simulink model "servo_dc_motor_sim_model"  (R2013b)
settings: Solver=ode45  StartTime=0.0  StopTime=0.6  RelTol=1e-3
libraries: powerlib x13, simulink x3, fl_lib x2
settings Model: Creator=User  LastModifiedBy=User
settings SolverCC: ZeroCrossControl=DisableAll

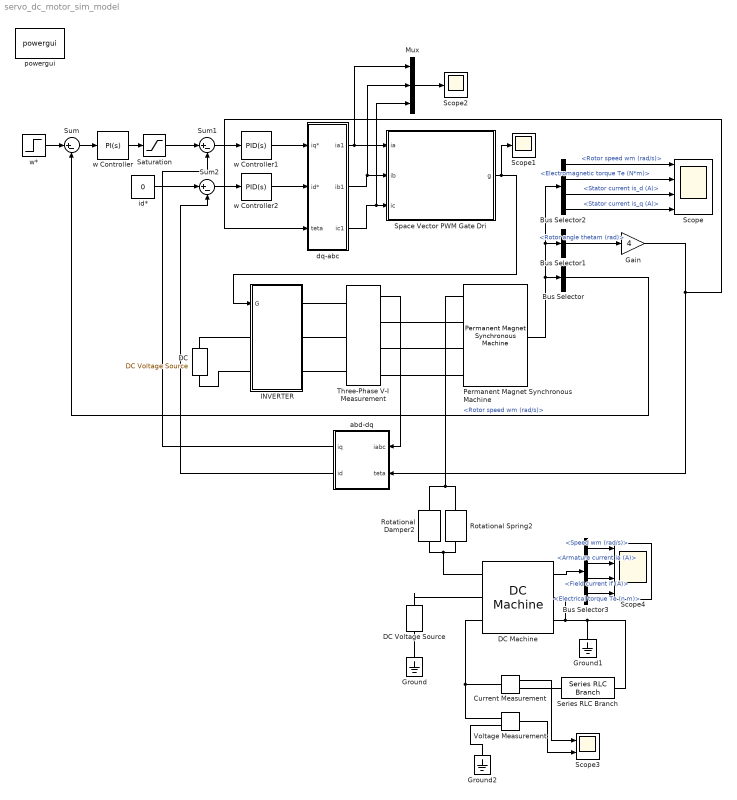
== system servo_dc_motor_sim_model ==
  Bus Selector : BusSelector  OutputSignals=Rotor speed wm (rad/s)
  Bus Selector1 : BusSelector  OutputSignals=Rotor angle thetam (rad)
  Bus Selector2 : BusSelector  OutputSignals=Rotor speed wm (rad/s),Electromagnetic torque Te (N*m),Stator current is_d (A),Stator current is_q (A)
  Bus Selector3 : BusSelector  OutputSignals=Speed wm (rad/s),Armature current ia (A),Field current if (A),Electrical torque Te (n m)
  Current Measurement : powerlib/Measurements/Current Measurement  PhasorSimulation=off  OutputType=Complex  PSBequivalent=0
  DC : powerlib/Electrical Sources/DC Voltage Source  Amplitude=400  Measurements=None
  DC Machine : powerlib/Machines/DC Machine  PresetModel=No  MechanicalLoad=Mechanical rotational port  FieldType=Wound  ShowDetailedParameters=on  RLa=[6.3 0.12]  RLf="[ 10.5  12]"  Laf=1.8  MachineConstant=Torque constant (N.m/A)  Ke=1.8  Kt=1.8  J=1  Bm=0  Tf=0  w0=1  Ifinit=1  TsPowergui=0  TsBlock=-1
  DC Voltage Source : powerlib/Electrical Sources/DC Voltage Source  Amplitude=12  Measurements=None
  Gain : Gain  Gain=4
  Ground : powerlib/Elements/Ground  LConnTagsString=a
  Ground1 : powerlib/Elements/Ground  LConnTagsString=a
  Ground2 : powerlib/Elements/Ground  LConnTagsString=a
  INVERTER : Subsystem
  Mux : Mux  Inputs=3
  Permanent Magnet Synchronous Machine : powerlib/Machines/Permanent Magnet Synchronous Machine  NbPhases=3  FluxDistribution=Sinusoidal  RotorType=Salient-pole  MechanicalLoad=Mechanical rotational port  PresetModel=No  ShowDetailedParameters=on  Resistance=0.61  Inductance=8.5e-3  dqInductances=[9.1e-3,11.5e-3]  La=0.000835  MachineConstant=Flux linkage established by magnets (V.s)  Flux=0.175  VoltageCst=126.966  TorqueCst=1.05  Flat=120  Mechanical=[0.0027 0.0004924 4 0]  PolePairs=4  InitialConditions=[0,0, 0,0]  InitialConditions5ph=[0 0 0 0 0 0]  TsPowergui=0  TsBlock=-1  RefAngle=90 degrees behind phase A axis (modified Park)
  Rotational Damper2 : fl_lib/Mechanical/Rotational Elements/Rotational Damper  D=1 N*m/(rad/s)  t_Log=off  w_Log=off  LocalVarNames=|t|w  LocalVarDescs=|t|w  LocalVarLogging=[0 0]
  Rotational Spring2 : fl_lib/Mechanical/Rotational Elements/Rotational Spring  spr_rate=5 N*m/rad  init_def=0 rad  t_Log=off  w_Log=off  phi_Log=off  LocalVarNames=|t|w|phi  LocalVarDescs=|t|w|phi  LocalVarLogging=[0 0 0]
  Saturation : Saturate  UpperLimit=20  LowerLimit=-20
  Scope : Scope  NumInputPorts=4
      settings: YMin=10~-25~-0.5~-20  YMax=110~25~7~20
  Scope1 : Scope
  Scope2 : Scope
      settings: YMin=-200  YMax=175  SaveName=ScopeData2
  Scope3 : Scope  NumInputPorts=2
      settings: YMin=-200~-5  YMax=175~5  SaveName=ScopeData5
  Scope4 : Scope  NumInputPorts=4
      settings: YMin=10~-25~-0.5~-20  YMax=110~25~7~20  SaveName=ScopeData6
  Series RLC Branch : powerlib/Elements/Series RLC Branch  LConnTagsString=__new0  RConnTagsString=__new0  BranchType=R  Resistance=20  Inductance=1e-3  SetiL0=off  InitialCurrent=0  Capacitance=1e-6  Setx0=off  InitialVoltage=0  Measurements=Branch voltage and current
  Space Vector PWM Gate Dri : Subsystem
  Sum : Sum  Inputs=|+-
  Sum1 : Sum  Inputs=|+-
  Sum2 : Sum  Inputs=|+-
  Three-Phase V-I Measurement : powerlib/Measurements/Three-Phase V-I Measurement  VoltageMeasurement=no  SetLabelV=off  LabelV=Vabc  Vpu=off  VpuLL=off  CurrentMeasurement=yes  SetLabelI=off  LabelI=Iabc  Ipu=off  Pbase=100e6  Vbase=500e3  OutputType=Complex  PhasorSimulation=off  PSBequivalent=0
  Voltage Measurement : powerlib/Measurements/Voltage Measurement  PhasorSimulation=off  OutputType=Complex  PSBequivalent=0
  abd-dq : Subsystem
  dq-abc : Subsystem
  id* : Constant  Value=0
  powergui : powerlib/powergui  Priority=1  SimulationMode=Continuous  SolverType=Tustin  SampleTime=50e-6  frequency=60  SPID=off  DisableSnubberDevices=off  DisableRonSwitches=off  DisableVfSwitches=off  SwTol=0  Interpol=off  DisplayEquations=off  frequencyindice=0  Pbase=100e6  ErrMax=1e-4  Iterations=50  UnitsV=kV  UnitsW=MW  FunctionMessages=off  echomessages=off  HookPort=off  EnableUseOfTLC=off  x0status=blocks  RestoreLinks=warning  ResistiveCurrentMeasurement=off  Frange=[0:2:500]  Ylog=off  Xlog=on  ShowGrid=off  save=off  variable=ZData  structure=ScopeData2  ZoomFFT=on  StartTime=0.05  cycles=10  DisplayStyle=1  fundamental=64.29  FreqAxis=on  MaxFrequency=1000  frequencyindicesteady=1  RmsSteady=1  display=off  Ts=0  methode=off
  w Controller : simulink/Continuous/PID Controller  Controller=PI  TimeDomain=Continuous-time  SampleTime=1  IntegratorMethod=Forward Euler  FilterMethod=Forward Euler  Form=Parallel  P=12  I=5  D=0  N=100  InitialConditionSource=internal  InitialConditionForIntegrator=0  InitialConditionForFilter=0  ExternalReset=none  LimitOutput=off  UpperSaturationLimit=inf  LowerSaturationLimit=-inf  LinearizeAsGain=on  AntiWindupMode=none  Kb=1  TrackingMode=off  Kt=1  PParamMin=[]  PParamMax=[]  IParamMin=[]  IParamMax=[]  DParamMin=[]  DParamMax=[]  NParamMin=[]  NParamMax=[]  KbParamMin=[]  KbParamMax=[]  KtParamMin=[]  KtParamMax=[]  POutMin=[]  POutMax=[]  IOutMin=[]  IOutMax=[]  DOutMin=[]  DOutMax=[]  NOutMin=[]  NOutMax=[]  KbOutMin=[]  KbOutMax=[]  KtOutMin=[]  KtOutMax=[]  IntegratorOutMin=[]  IntegratorOutMax=[]  FilterOutMin=[]  FilterOutMax=[]  SumOutMin=[]  SumOutMax=[]  SumI1OutMin=[]  SumI1OutMax=[]  SumI2OutMin=[]  SumI2OutMax=[]  SumI3OutMin=[]  SumI3OutMax=[]  SumDOutMin=[]  SumDOutMax=[]  SaturationOutMin=[]  SaturationOutMax=[]  IntegratorContinuousStateAttributes=''  IntegratorStateMustResolveToSignalObject=off  IntegratorRTWStateStorageClass=Auto  FilterContinuousStateAttributes=''  FilterStateMustResolveToSignalObject=off  FilterRTWStateStorageClass=Auto
  w Controller1 : simulink/Continuous/PID Controller  Controller=PID  TimeDomain=Continuous-time  SampleTime=1  IntegratorMethod=Forward Euler  FilterMethod=Forward Euler  Form=Parallel  P=5  I=12  D=5  N=100  InitialConditionSource=internal  InitialConditionForIntegrator=0  InitialConditionForFilter=0  ExternalReset=none  LimitOutput=off  UpperSaturationLimit=inf  LowerSaturationLimit=-inf  LinearizeAsGain=on  AntiWindupMode=none  Kb=1  TrackingMode=off  Kt=1  PParamMin=[]  PParamMax=[]  IParamMin=[]  IParamMax=[]  DParamMin=[]  DParamMax=[]  NParamMin=[]  NParamMax=[]  KbParamMin=[]  KbParamMax=[]  KtParamMin=[]  KtParamMax=[]  POutMin=[]  POutMax=[]  IOutMin=[]  IOutMax=[]  DOutMin=[]  DOutMax=[]  NOutMin=[]  NOutMax=[]  KbOutMin=[]  KbOutMax=[]  KtOutMin=[]  KtOutMax=[]  IntegratorOutMin=[]  IntegratorOutMax=[]  FilterOutMin=[]  FilterOutMax=[]  SumOutMin=[]  SumOutMax=[]  SumI1OutMin=[]  SumI1OutMax=[]  SumI2OutMin=[]  SumI2OutMax=[]  SumI3OutMin=[]  SumI3OutMax=[]  SumDOutMin=[]  SumDOutMax=[]  SaturationOutMin=[]  SaturationOutMax=[]  IntegratorContinuousStateAttributes=''  IntegratorStateMustResolveToSignalObject=off  IntegratorRTWStateStorageClass=Auto  FilterContinuousStateAttributes=''  FilterStateMustResolveToSignalObject=off  FilterRTWStateStorageClass=Auto
  w Controller2 : simulink/Continuous/PID Controller  Controller=PID  TimeDomain=Continuous-time  SampleTime=1  IntegratorMethod=Forward Euler  FilterMethod=Forward Euler  Form=Parallel  P=16  I=5  D=5  N=100  InitialConditionSource=internal  InitialConditionForIntegrator=0  InitialConditionForFilter=0  ExternalReset=none  LimitOutput=off  UpperSaturationLimit=inf  LowerSaturationLimit=-inf  LinearizeAsGain=on  AntiWindupMode=none  Kb=1  TrackingMode=off  Kt=1  PParamMin=[]  PParamMax=[]  IParamMin=[]  IParamMax=[]  DParamMin=[]  DParamMax=[]  NParamMin=[]  NParamMax=[]  KbParamMin=[]  KbParamMax=[]  KtParamMin=[]  KtParamMax=[]  POutMin=[]  POutMax=[]  IOutMin=[]  IOutMax=[]  DOutMin=[]  DOutMax=[]  NOutMin=[]  NOutMax=[]  KbOutMin=[]  KbOutMax=[]  KtOutMin=[]  KtOutMax=[]  IntegratorOutMin=[]  IntegratorOutMax=[]  FilterOutMin=[]  FilterOutMax=[]  SumOutMin=[]  SumOutMax=[]  SumI1OutMin=[]  SumI1OutMax=[]  SumI2OutMin=[]  SumI2OutMax=[]  SumI3OutMin=[]  SumI3OutMax=[]  SumDOutMin=[]  SumDOutMax=[]  SaturationOutMin=[]  SaturationOutMax=[]  IntegratorContinuousStateAttributes=''  IntegratorStateMustResolveToSignalObject=off  IntegratorRTWStateStorageClass=Auto  FilterContinuousStateAttributes=''  FilterStateMustResolveToSignalObject=off  FilterRTWStateStorageClass=Auto
  w* : Step  Time=0.3  Before=100  After=-100  SampleTime=0
  wires:
  Sum/1 -> w Controller/1
  w*/1 -> Sum/1
  Permanent Magnet Synchronous Machine/1 -> Bus Selector/1, Bus Selector1/1, Bus Selector2/1
  Bus Selector/1 -> Sum/2  "<Rotor speed wm (rad/s)>"
  Bus Selector1/1 -> Gain/1  "<Rotor angle thetam (rad)>"
  Bus Selector2/1 -> Scope/1  "<Rotor speed wm (rad/s)>"
  Bus Selector2/2 -> Scope/2  "<Electromagnetic torque Te (N*m)>"
  Bus Selector2/3 -> Scope/3  "<Stator current is_d (A)>"
  Bus Selector2/4 -> Scope/4  "<Stator current is_q (A)>"
  w Controller/1 -> Saturation/1
  Sum1/1 -> w Controller1/1
  w Controller1/1 -> dq-abc/1(iq*)
  id*/1 -> Sum2/1
  Sum2/1 -> w Controller2/1
  w Controller2/1 -> dq-abc/2(id*)
  Gain/1 -> abd-dq/2(teta), dq-abc/3(teta)
  Three-Phase V-I Measurement/1 -> abd-dq/1(iabc)
  abd-dq/1(iq) -> Sum1/2
  abd-dq/2(id) -> Sum2/2
  dq-abc/1(ia1) -> Mux/1, Space Vector PWM Gate Dri/1(ia)
  dq-abc/2(ib1) -> Mux/2, Space Vector PWM Gate Dri/2(ib)
  dq-abc/3(ic1) -> Mux/3, Space Vector PWM Gate Dri/3(ic)
  Space Vector PWM Gate Dri/1(g) -> INVERTER/1(G), Scope1/1
  Mux/1 -> Scope2/1
  Saturation/1 -> Sum1/1
  Current Measurement/1 -> Scope3/1
  Voltage Measurement/1 -> Scope3/2
  DC Machine/1 -> Bus Selector3/1
  Bus Selector3/1 -> Scope4/1  "<Speed wm (rad/s)>"
  Bus Selector3/2 -> Scope4/2  "<Armature current ia (A)>"
  Bus Selector3/3 -> Scope4/3  "<Field current if (A)>"
  Bus Selector3/4 -> Scope4/4  "<Electrical torque Te (n m)>"
  connections:
  Three-Phase V-I Measurement/LConn1 -- INVERTER/RConn1
  Three-Phase V-I Measurement/LConn2 -- INVERTER/RConn2
  Three-Phase V-I Measurement/LConn3 -- INVERTER/RConn3
  Three-Phase V-I Measurement/RConn1 -- Permanent Magnet Synchronous Machine/LConn2
  Three-Phase V-I Measurement/RConn2 -- Permanent Magnet Synchronous Machine/LConn3
  Three-Phase V-I Measurement/RConn3 -- Permanent Magnet Synchronous Machine/LConn4
  DC/RConn1 -- INVERTER/LConn1
  DC/LConn1 -- INVERTER/LConn2
  Rotational Spring2/RConn1 -- DC Machine/LConn1 -- Rotational Damper2/RConn1
  Rotational Damper2/LConn1 -- Permanent Magnet Synchronous Machine/LConn1 -- Rotational Spring2/LConn1
  DC Voltage Source/RConn1 -- DC Machine/LConn2
  Ground/LConn1 -- DC Voltage Source/LConn1
  Series RLC Branch/RConn1 -- DC Machine/RConn1 -- DC Machine/RConn2 -- Ground1/LConn1
  Current Measurement/RConn1 -- Series RLC Branch/LConn1
  DC Machine/LConn3 -- Voltage Measurement/LConn1 -- Current Measurement/LConn1
  Voltage Measurement/LConn2 -- Ground2/LConn1

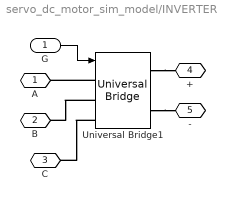
== system servo_dc_motor_sim_model/INVERTER ==
  G : Inport
  Universal Bridge1 : powerlib/Power Electronics/Universal Bridge  Arms=3  SnubberResistance=1e5  SnubberCapacitance=inf  Device=IGBT / Diodes  Ron=1e-3  Lon=0  ForwardVoltages="[  0  0  ]"  ForwardVoltage=0  GTOparameters=[ 10e-6 , 20e-6 ]  IGBTparameters=[ 1e-6 , 2e-6 ]  Measurements=None  Measurements_2=None  converterType=Rectifier
  A : PMIOPort  Port=1  Side=Right
  B : PMIOPort  Port=2  Side=Right
  C : PMIOPort  Port=3  Side=Right
  + : PMIOPort  Port=4  Side=Left
  - : PMIOPort  Port=5  Side=Left
  wires:
  G/1 -> Universal Bridge1/1
  connections:
  Universal Bridge1/RConn2 -- -/RConn1
  Universal Bridge1/RConn1 -- +/RConn1
  Universal Bridge1/LConn3 -- C/RConn1
  Universal Bridge1/LConn2 -- B/RConn1
  Universal Bridge1/LConn1 -- A/RConn1

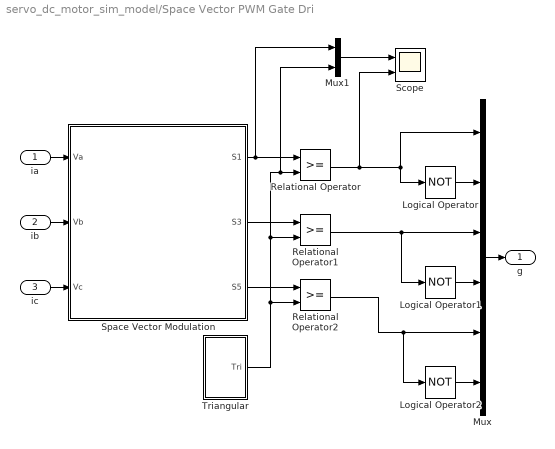
== system servo_dc_motor_sim_model/Space Vector PWM Gate Dri ==
  ia : Inport
  ib : Inport  Port=2
  ic : Inport  Port=3
  Logical Operator : Logic  Operator=NOT  AllPortsSameDT=off  OutDataTypeStr=boolean
  Logical Operator1 : Logic  Operator=NOT  AllPortsSameDT=off  OutDataTypeStr=boolean
  Logical Operator2 : Logic  Operator=NOT  AllPortsSameDT=off  OutDataTypeStr=boolean
  Mux : Mux  Inputs=6
  Mux1 : Mux  Inputs=2
  Relational Operator : RelationalOperator  OutDataTypeStr=boolean
  Relational Operator1 : RelationalOperator  OutDataTypeStr=boolean
  Relational Operator2 : RelationalOperator  OutDataTypeStr=boolean
  Scope : Scope  NumInputPorts=2
      settings: YMin=-0.05~0.95  YMax=1.05~1.05  SaveName=ScopeData4
  Space Vector Modulation : Subsystem
  Triangular : Subsystem
  g : Outport
  wires:
  Logical Operator/1 -> Mux/2
  Relational Operator1/1 -> Logical Operator1/1, Mux/3
  Triangular/1(Tri) -> Relational Operator2/2, Relational Operator1/2, Mux1/2, Relational Operator/2
  Space Vector Modulation/1(S1) -> Mux1/1, Relational Operator/1
  Space Vector Modulation/2(S3) -> Relational Operator1/1
  Space Vector Modulation/3(S5) -> Relational Operator2/1
  Mux/1 -> g/1
  Relational Operator/1 -> Scope/2, Logical Operator/1, Mux/1
  ia/1 -> Space Vector Modulation/1(Va)
  Logical Operator1/1 -> Mux/4
  Logical Operator2/1 -> Mux/6
  Relational Operator2/1 -> Logical Operator2/1, Mux/5
  ib/1 -> Space Vector Modulation/2(Vb)
  ic/1 -> Space Vector Modulation/3(Vc)
  Mux1/1 -> Scope/1

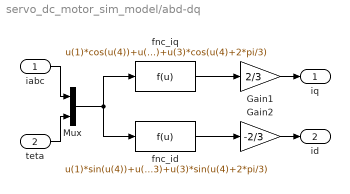
== system servo_dc_motor_sim_model/abd-dq ==
  iabc : Inport
  teta : Inport  Port=2
  Gain1 : Gain  Gain=2/3
  Gain2 : Gain  Gain=-2/3
  Mux : Mux  Inputs=2
  fnc_id : Fcn  Expr=u(1)*sin(u(4))+u(2)*sin(u(4)-2*pi/3)+u(3)*sin(u(4)+2*pi/3)
  fnc_iq : Fcn  Expr=u(1)*cos(u(4))+u(2)*cos(u(4)-2*pi/3)+u(3)*cos(u(4)+2*pi/3)
  iq : Outport
  id : Outport  Port=2
  wires:
  fnc_id/1 -> Gain2/1
  Gain1/1 -> iq/1
  teta/1 -> Mux/2
  iabc/1 -> Mux/1
  Mux/1 -> fnc_iq/1, fnc_id/1
  Gain2/1 -> id/1
  fnc_iq/1 -> Gain1/1

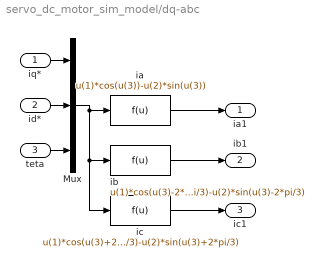
== system servo_dc_motor_sim_model/dq-abc ==
  iq* : Inport
  id* : Inport  Port=2
  teta : Inport  Port=3
  Mux : Mux  Inputs=3
  ia : Fcn  Expr=u(1)*cos(u(3))-u(2)*sin(u(3))
  ib : Fcn  Expr=u(1)*cos(u(3)-2*pi/3)-u(2)*sin(u(3)-2*pi/3)
  ic : Fcn  Expr=u(1)*cos(u(3)+2*pi/3)-u(2)*sin(u(3)+2*pi/3)
  ia1 : Outport
  ib1 : Outport  Port=2
  ic1 : Outport  Port=3
  wires:
  id*/1 -> Mux/2
  ia/1 -> ia1/1
  ib/1 -> ib1/1
  teta/1 -> Mux/3
  ic/1 -> ic1/1
  iq*/1 -> Mux/1
  Mux/1 -> ic/1, ib/1, ia/1

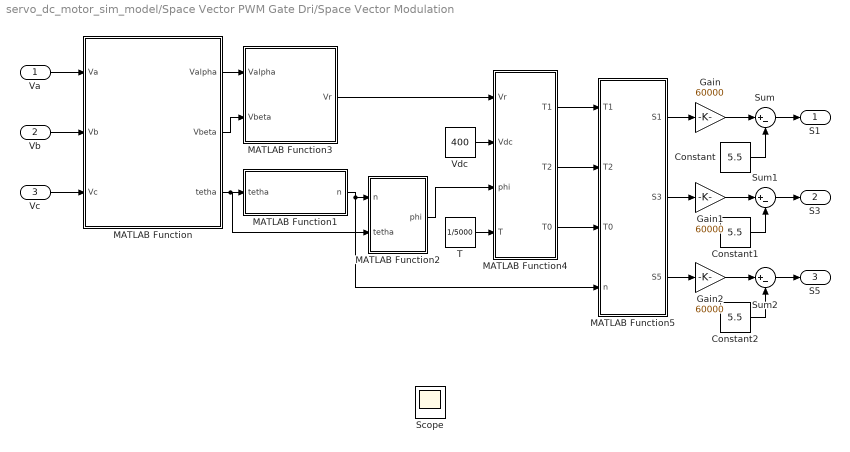
== system servo_dc_motor_sim_model/Space Vector PWM Gate Dri/Space Vector Modulation ==
  Va : Inport
  Vb : Inport  Port=2
  Vc : Inport  Port=3
  Constant : Constant  Value=5.5
  Constant1 : Constant  Value=5.5
  Constant2 : Constant  Value=5.5
  Gain : Gain  Gain=60000
  Gain1 : Gain  Gain=60000
  Gain2 : Gain  Gain=60000
  MATLAB Function : MATLAB Function  TreatAsAtomicUnit=on
  MATLAB Function1 : MATLAB Function  TreatAsAtomicUnit=on
  MATLAB Function2 : MATLAB Function  TreatAsAtomicUnit=on
  MATLAB Function3 : MATLAB Function  TreatAsAtomicUnit=on
  MATLAB Function4 : MATLAB Function  TreatAsAtomicUnit=on
  MATLAB Function5 : MATLAB Function  TreatAsAtomicUnit=on
  Scope : Scope
      settings: SaveName=ScopeData3
  Sum : Sum  Inputs=|+-
  Sum1 : Sum  Inputs=|+-
  Sum2 : Sum  Inputs=|+-
  T : Constant  Value=1/5000
  Vdc : Constant  Value=400
  S1 : Outport
  S3 : Outport  Port=2
  S5 : Outport  Port=3
  wires:
  MATLAB Function4/1(T1) -> MATLAB Function5/1(T1)
  MATLAB Function5/3(S5) -> Gain2/1
  MATLAB Function5/1(S1) -> Gain/1
  MATLAB Function4/2(T2) -> MATLAB Function5/2(T2)
  MATLAB Function4/3(T0) -> MATLAB Function5/3(T0)
  Va/1 -> MATLAB Function/1(Va)
  Vc/1 -> MATLAB Function/3(Vc)
  Vb/1 -> MATLAB Function/2(Vb)
  MATLAB Function/3(tetha) -> MATLAB Function2/2(tetha), MATLAB Function1/1(tetha)
  MATLAB Function1/1(n) -> MATLAB Function5/4(n), MATLAB Function2/1(n)
  MATLAB Function/1(Valpha) -> MATLAB Function3/1(Valpha)
  MATLAB Function/2(Vbeta) -> MATLAB Function3/2(Vbeta)
  MATLAB Function2/1(phi) -> MATLAB Function4/3(phi)
  MATLAB Function3/1(Vr) -> MATLAB Function4/1(Vr)
  Vdc/1 -> MATLAB Function4/2(Vdc)
  T/1 -> MATLAB Function4/4(T)
  MATLAB Function5/2(S3) -> Gain1/1
  Constant/1 -> Sum/2
  Gain/1 -> Sum/1
  Sum/1 -> S1/1
  Constant2/1 -> Sum2/2
  Constant1/1 -> Sum1/2
  Gain1/1 -> Sum1/1
  Sum1/1 -> S3/1
  Sum2/1 -> S5/1
  Gain2/1 -> Sum2/1

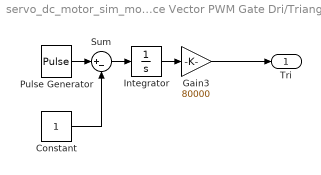
== system servo_dc_motor_sim_model/Space Vector PWM Gate Dri/Triangular ==
  Constant : Constant
  Gain3 : Gain  Gain=80000
  Integrator : Integrator
  Pulse Generator : DiscretePulseGenerator  PulseType=Time based  Amplitude=2  Period=1/40000  PulseWidth=50
  Sum : Sum  Inputs=|+-
  Tri : Outport
  wires:
  Sum/1 -> Integrator/1
  Pulse Generator/1 -> Sum/1
  Constant/1 -> Sum/2
  Gain3/1 -> Tri/1
  Integrator/1 -> Gain3/1

== matlab function servo_dc_motor_sim_model/Space Vector PWM Gate Dri/Space Vector Modulation/MATLAB Function1 ==
  data: tetha input; n output
function n = Sector(tetha)
n=0;
if (tetha>0)&(tetha<=pi/3)
    n=1;
end;
if (tetha>pi/3)&(tetha<=2*pi/3)
    n=2;
end;
if (tetha>2*pi/3)&(tetha<=pi)
    n=3;
end;
if (tetha<=-2*pi/3)&(tetha>-pi)
    n=4;
end;
if (tetha<=-pi/3)&(tetha>-2*pi/3)
    n=5;
end;
if (tetha<=0)&(tetha>-pi/3)
    n=6;
end;

== matlab function servo_dc_motor_sim_model/Space Vector PWM Gate Dri/Space Vector Modulation/MATLAB Function ==
  data: Va input; Valpha output; Vb input; Vc input; Vbeta output; tetha output
function [Valpha, Vbeta, tetha] = clark(Va, Vb, Vc)
Valpha=Va-Vb/2-Vc/2;
Vbeta=sqrt(3)/2*(Vb-Vc);
tetha=atan2(Vbeta,Valpha);

== matlab function servo_dc_motor_sim_model/Space Vector PWM Gate Dri/Space Vector Modulation/MATLAB Function2 ==
  data: n input; phi output; tetha input
function phi = Phi(n,tetha)
phi=0;
if (n==1)
    phi=tetha;
end;
if (n==2)
    phi=tetha-pi/3;
end;
if (n==3)
    phi=tetha-2*pi/3;
end;
if (n==4)
    phi=pi+tetha;
end;
if (n==5)
    phi=2*pi/3+tetha;
end;
if (n==6)
    phi=pi/3+tetha;
end;

== matlab function servo_dc_motor_sim_model/Space Vector PWM Gate Dri/Space Vector Modulation/MATLAB Function3 ==
  data: Valpha input; Vr output; Vbeta input
function Vr = Vref(Valpha,Vbeta)
Vr=sqrt(Valpha^2+Vbeta^2);

== matlab function servo_dc_motor_sim_model/Space Vector PWM Gate Dri/Space Vector Modulation/MATLAB Function4 ==
  data: Vr input; T1 output; Vdc input; phi input; T input; T2 output; T0 output
function [T1,T2,T0] = Timing(Vr,Vdc,phi,T)
x=Vr/Vdc;
T1=T*x*sin(pi/3-phi)/sin(pi/3);
T2=T*x*sin(phi)/sin(pi/3);
T0=T-T1-T2;

== matlab function servo_dc_motor_sim_model/Space Vector PWM Gate Dri/Space Vector Modulation/MATLAB Function5 ==
  data: T1 input; T2 input; T0 input; S1 output; n input; S3 output; S5 output
function [S1,S3,S5] = GATE(T1,T2,T0,n)
S1=0;
S3=0;
S5=0;
if(n==1)
    S1=T1+T2+T0/2;
    S3=T2+T0/2;
    S5=T0/2;
end;
if(n==2)
    S1=T1+T0/2;
    S3=T1+T2+T0/2;
    S5=T0/2;
end;
if(n==3)
    S1=T0/2;
    S3=T1+T2+T0/2;
    S5=T2+T0/2;
end;
if(n==4)
    S1=T0/2;
    S3=T1+T0/2;
    S5=T1+T2+T0/2;
end;
if(n==5)
    S1=T2+T0/2;
    S3=T0/2;
    S5=T1+T2+T0/2;
end;
if(n==6)
    S1=T1+T2+T0/2;
    S3=T0/2;
    S5=T1+T0/2;
end;
